simulink model "plant4_ieee"  (R2015a)
settings: Solver=ode23s  StartTime=0.0  StopTime=3  RelTol=1e-3
values from neighbouring files (symbols this model uses):
  A = [2.15382349002 0.214572825654 1.88950096566 -0.29867853041 0.113062196229 -1.01325242733 0.619436209547 2.86203861181 4.48591725582 -0.687413149535 3.93984391159 1.51814076611 ... (36 elements, 6x6)]    [De2.mat]    (also in main_elca.m = [   -2.1     0.3     0.5     0.9; main_elca_nonsquare.m = [-31.31 0 -2.833e4;0 -10.25 8001;1 -1 0]; main_elca_siso.m = [-31.31 0 -2.833e4;0 -10.25 8001;1 -1 0]; main_elca_siso_conference.m = [-31.31 0 -2.833e4;0 -10.25 8001;1 -1 0])
  Af = -Bfi*Cfi*eye(size(B,2))    [main_c.m]    (also in main_elca.m; main_elca_nonsquare.m; main_elca_siso.m; main_elca_siso_conference.m)
  B = [-3.59754701628 1.03900107164 -0.0588288788819 1.91030576689 -0.469593029649 2.39038747798 -2.63971513379 2.37119746965 -0.382769327239 -1.07761123079 -0.524364953631 2.34772297005 ... (18 elements, 6x3)]    [De2.mat]    (also in main_elca.m = [   1   -0.4; main_elca_nonsquare.m = [28.06 0 0]'; main_elca_siso.m = [28.06 0 0]'; main_elca_siso_conference.m = [28.06;0;0])
  Bf = Bfi*eye(size(B,2))    [main_c.m]    (also in main_elca.m; main_elca_nonsquare.m; main_elca_siso.m; main_elca_siso_conference.m)
  C = [2.23974909489  -2.89672334174  -0.970355173176  -2.60836731796  -0.958327072966  -1.82597470965; -0.233950036489  3.17111373121  -0.953917376412  0.311760155602  0.255404296822  2.81333280658]    [De2.mat]    (also in main_elca.m = [2  -2  -1   4; main_elca_nonsquare.m = [1 0 0]; main_elca_siso.m = [1 0 0]; main_elca_siso_conference.m = [1 0 0])
  Ced = inv(Re)*Be_aug'*inv((Ae_aug-Be_aug*Ke)')*Pe_aug    [main_elca.m]    (also in main_elca_nonsquare.m; main_elca_siso.m; main_elca_siso_conference.m; main_elca_siso_luenberger.m)
  Cf = Cfi*eye(size(B,2))    [main_c.m]    (also in main_elca.m; main_elca_nonsquare.m; main_elca_siso.m; main_elca_siso_conference.m)
  D = [0  0  0; 0  0  0]    [De2.mat]    (also in main_c.m = zeros(p,m); main_elca.m = zeros(p,m); main_elca_nonsquare.m = zeros(p,m); main_elca_siso.m = zeros(p,m))
  De = [0.318518810679  1.43017682461; 1.54076970526  2.04306947136; -0.541765795745  0.784935731305; 0.271599502383  0.685376596238; -1.34549150719  -1.13203605501; -1.47309738777  -1.64908854438]    [De2.mat]    (also in De_.mat; De_conference.mat = [-1.1479527789  -0.666890670701; 0.104874716016  0.187331024; De_term.mat; generate_De.m = randn(n,p))
  de_aug_b = J*C_tilde*B    [main_elca.m]    (also in main_elca_nonsquare.m; main_elca_siso.m; main_elca_siso_conference.m; main_elca_siso_luenberger.m)
  Ec = -inv(R_bar)*( ( C - D*Kc )*inv( A - B*Kc )*B - D )'*Qc    [TZOCS.m]    (also in main_c.m = -inv(R_bar)*( ( C_aug - D_aug*Kc )*inv( A_aug - B_aug*Kc )*B; main_elca.m = -inv(R_bar)*( ( C_aug - D_aug*Kc )*inv( A_aug - B_aug*Kc )*B; main_elca_nonsquare.m = -inv(R_bar)*( ( C_aug - D_aug*Kc )*inv( A_aug - B_aug*Kc )*B; main_elca_siso.m = -inv(R_bar)*( ( C_aug - D_aug*Kc )*inv( A_aug - B_aug*Kc )*B)
  Ee = -inv(Re)*( ( Ce_aug )*inv( Ae_aug - Be_aug*Ke )*Be_aug )'*Qe    [main_c.m]    (also in main_elca.m; main_elca_nonsquare.m; main_elca_siso.m; main_elca_siso_conference.m)
  eta = 0.532094499421    [eta value.mat]    (also in eta_value.mat = [-2.43750362486  -7.92336865107; -8.9760065871  -9.529746909; generate_eta.m = (1*randn(p,p)); main_c.m = 10*eta; main_elca_nonsquare.m = eye(1))
  Kc1 = Kc(:,1:n)    [main_c.m]    (also in main_elca.m; main_elca_nonsquare.m; main_elca_siso.m; main_elca_siso_conference.m)
  Kc2 = Kc(:,n+1:end)    [main_c.m]    (also in main_elca.m; main_elca_nonsquare.m; main_elca_siso.m; main_elca_siso_conference.m)
  Kd_1 = Kd(1,1)    [main_c.m]    (also in main_elca.m; main_elca_nonsquare.m; main_elca_siso.m; main_elca_siso_conference.m)
  Ke1 = Ke(:,1:n)    [main_c.m]    (also in main_elca.m; main_elca_nonsquare.m; main_elca_siso.m; main_elca_siso_conference.m)
  Ke2 = Ke(:,n+1:end)    [main_c.m]    (also in main_elca.m; main_elca_nonsquare.m; main_elca_siso.m; main_elca_siso_conference.m)
  Ki_1 = Ki(1,1)    [main_c.m]    (also in main_elca.m; main_elca_nonsquare.m; main_elca_siso.m; main_elca_siso_conference.m)
  Kp_1 = Kp(1,1)    [main_c.m]    (also in main_elca.m; main_elca_nonsquare.m; main_elca_siso.m; main_elca_siso_conference.m)
settings Model: Creator=Elca  LastModifiedBy=Elca

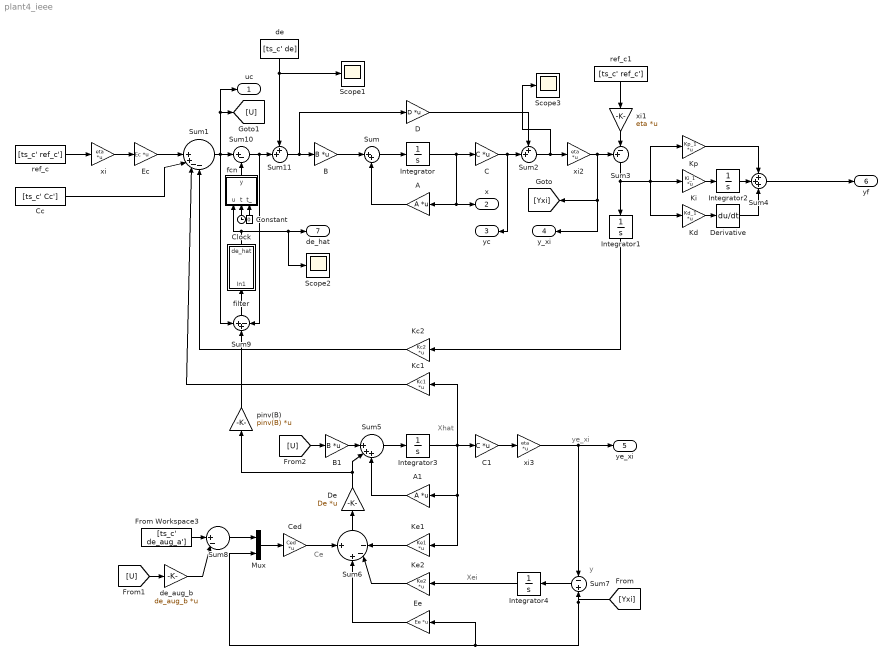
== system plant4_ieee ==
  note: Ce
  note: Xhat
  note: Xei
  note: ye_xi
  note: y
  A : Gain  Gain=A  Multiplication=Matrix(K*u)
  A1 : Gain  Gain=A  Multiplication=Matrix(K*u)
  B : Gain  Gain=B  Multiplication=Matrix(K*u)
  B1 : Gain  Gain=B  Multiplication=Matrix(K*u)
  C : Gain  Gain=C  Multiplication=Matrix(K*u)
  C1 : Gain  Gain=C  Multiplication=Matrix(K*u)
  Cc : FromWorkspace  VariableName=[ts_c' Cc']  SampleTime=0
  Ced : Gain  Gain=Ced  Multiplication=Matrix(K*u)
  Clock : Clock
  Constant : Constant  Value=0
  D : Gain  Gain=D  Multiplication=Matrix(K*u)
  De : Gain  Gain=De  Multiplication=Matrix(K*u)
  Derivative : Derivative
  Ec : Gain  Gain=Ec  Multiplication=Matrix(K*u)
  Ee : Gain  Gain=Ee  Multiplication=Matrix(K*u)
  From Workspace3 : FromWorkspace  VariableName=[ts_c' de_aug_a']  SampleTime=0
  Integrator{,1..2,4} (4 alike) : Integrator
  Integrator3 : Integrator  InitialCondition=0.1
  Kc1 : Gain  Gain=Kc1  Multiplication=Matrix(K*u)
  Kc2 : Gain  Gain=Kc2  Multiplication=Matrix(K*u)
  Kd : Gain  Gain=Kd_1  Multiplication=Matrix(K*u)
  Ke1 : Gain  Gain=Ke1  Multiplication=Matrix(K*u)
  Ke2 : Gain  Gain=Ke2  Multiplication=Matrix(K*u)
  Ki : Gain  Gain=Ki_1  Multiplication=Matrix(K*u)
  Kp : Gain  Gain=Kp_1  Multiplication=Matrix(K*u)
  Mux : Mux  Inputs=2
  Scope1 : Scope
      settings: YMin=-100  YMax=100
  Scope2 : Scope
      settings: TimeRange=3  YMin=1.48131  YMax=1.48131
  Scope3 : Scope
      settings: YMin=-3e+286  YMax=2.5e+285  SaveName=ScopeData2
  Sum : Sum  Inputs=|++
  Sum1 : Sum  Inputs=|||++--
  Sum10 : Sum  Inputs=|+-
  Sum11 : Sum  Inputs=++|
  Sum2 : Sum  Inputs=++|
  Sum3 : Sum  Inputs=+-|
  Sum4 : Sum  Inputs=+++
  Sum5 : Sum  Inputs=||+++
  Sum6 : Sum  Inputs=+|+--
  Sum7 : Sum  Inputs=-+
  Sum8 : Sum  Inputs=||+-|
  Sum9 : Sum  Inputs=++-
  de : FromWorkspace  VariableName=[ts_c' de]  SampleTime=0
  de_aug_b : Gain  Gain=de_aug_b  Multiplication=Matrix(K*u)
  fcn : MATLAB Function  TreatAsAtomicUnit=on
  filter : Subsystem
  pinv(B) : Gain  Gain=pinv(B)  Multiplication=Matrix(K*u)
  ref_c : FromWorkspace  VariableName=[ts_c' ref_c']  SampleTime=0
  ref_c1 : FromWorkspace  VariableName=[ts_c' ref_c']  SampleTime=0
  xi{,1..3} (4 alike) : Gain  Gain=eta  Multiplication=Matrix(K*u)
  uc : Outport  PortDimensions=m
  x : Outport  Port=2
  yc : Outport  Port=3
  y_xi : Outport  Port=4
  ye_xi : Outport  Port=5
  yf : Outport  Port=6
  de_hat : Outport  Port=7  PortDimensions=m
  wires:
  Ec/1 -> Sum1/1
  Integrator/1 -> x/1, A/1, C/1
  Sum2/1 -> Scope3/1, xi2/1
  C/1 -> yc/1, Sum2/2
  D/1 -> Sum2/1
  Sum/1 -> Integrator/1
  A/1 -> Sum/2
  B/1 -> Sum/1
  ref_c/1 -> xi/1
  Cc/1 -> Sum1/2
  xi2/1 -> y_xi/1, [Yxi], Sum3/1
  ref_c1/1 -> xi1/1
  Sum3/1 -> Kd/1, Kp/1, Ki/1, Integrator1/1
  xi/1 -> Ec/1
  xi1/1 -> Sum3/2
  Kd/1 -> Derivative/1
  Kp/1 -> Sum4/1
  Integrator2/1 -> Sum4/2
  Sum4/1 -> yf/1
  Derivative/1 -> Sum4/3
  Ki/1 -> Integrator2/1
  Sum5/1 -> Integrator3/1
  Integrator3/1 -> Ke1/1, A1/1, Kc1/1, C1/1
  A1/1 -> Sum5/3
  C1/1 -> xi3/1
  Integrator4/1 -> Ke2/1
  xi3/1 -> ye_xi/1, Sum7/1
  Mux/1 -> Ced/1
  [Yxi] -> Mux/2, Ee/1, Sum7/2
  [U] -> de_aug_b/1
  Integrator1/1 -> Kc2/1
  Sum7/1 -> Integrator4/1
  Ced/1 -> Sum6/1
  Sum6/1 -> De/1
  Ee/1 -> Sum6/2
  Ke2/1 -> Sum6/3
  Ke1/1 -> Sum6/4
  B1/1 -> Sum5/1
  De/1 -> pinv(B)/1, Sum5/2
  Kc2/1 -> Sum1/4
  [U] -> B1/1
  Sum8/1 -> Mux/1
  From Workspace3/1 -> Sum8/1
  de_aug_b/1 -> Sum8/2
  Kc1/1 -> Sum1/3
  pinv(B)/1 -> Sum9/2
  Sum9/1 -> filter/1(In1)
  filter/1(de_hat) -> de_hat/1, Scope2/1, fcn/1(u)
  Sum1/1 -> [U], uc/1, Sum9/1, Sum10/1
  Sum10/1 -> Sum9/3, Sum11/2
  Sum11/1 -> D/1, B/1
  de/1 -> Sum11/1, Scope1/1
  Clock/1 -> fcn/2(t)
  Constant/1 -> fcn/3(t_)
  fcn/1(y) -> Sum10/2

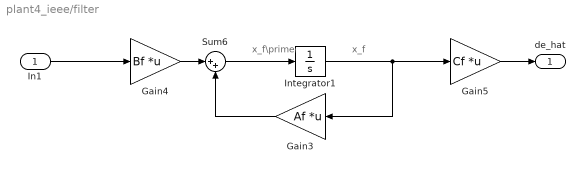
== system plant4_ieee/filter ==
  note: x_f\prime
  note: x_f
  In1 : Inport
  Gain3 : Gain  Gain=Af  Multiplication=Matrix(K*u)
  Gain4 : Gain  Gain=Bf  Multiplication=Matrix(K*u)
  Gain5 : Gain  Gain=Cf  Multiplication=Matrix(K*u)
  Integrator1 : Integrator
  Sum6 : Sum  Inputs=|++
  de_hat : Outport
  wires:
  Gain4/1 -> Sum6/1
  Sum6/1 -> Integrator1/1
  Integrator1/1 -> Gain3/1, Gain5/1
  Gain3/1 -> Sum6/2
  In1/1 -> Gain4/1
  Gain5/1 -> de_hat/1

== matlab function plant4_ieee/fcn ==
  data: u input; y output; t input; t_ input
function y = fcn(u,t,t_)
%#codegen
    if t > t_
        y = u;
    else
        y = 0*u;
    end
end
